simulink model "gm_lookupTable"  (R2019b)
settings: Solver=FixedStepAuto  StartTime=0.0  StopTime=0.01  RelTol=1e-3
libraries: hdlsllib x1
settings Model: Creator=bwieczorek  LastModifiedBy=bwieczorek
settings OptimizationCC: BlockReduction=off  ConditionallyExecuteInputs=off
settings DebuggingCC: SignalRangeChecking=warning  InheritedTsInSrcMsg=none

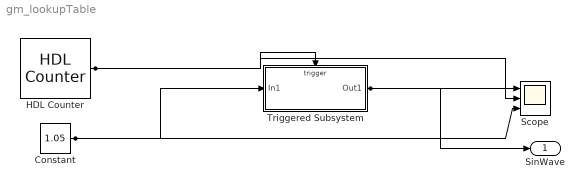
== system gm_lookupTable ==
  Constant : Constant  Value=1.05  OutDataTypeStr=fixdt(1,18,8)  SampleTime=1e-6
  HDL Counter : hdlsllib/Sources/HDL Counter  CountType=Count limited  CountInit=0  CountStep=1  CountMax=1  CountFromType=Initial value  CountFrom=0  CountResetPort=off  CountLoadPort=off  CountEnbPort=off  CountDirPort=off  CountDataType=Unsigned  CountWordLen=1  CountFracLen=0  CountSampTime=1e-6
      settings: SourceProductName=Simulink
  Scope : Scope  NumInputPorts=3
  Triggered Subsystem : Subsystem
  SinWave : Outport  VectorParamsAs1DForOutWhenUnconnected=off
  wires:
  Constant/1 -> Scope/3, Triggered Subsystem/1(In1)
  HDL Counter/1 -> Scope/2, Triggered Subsystem/Trigger
  Triggered Subsystem/1(Out1) -> Scope/1, SinWave/1

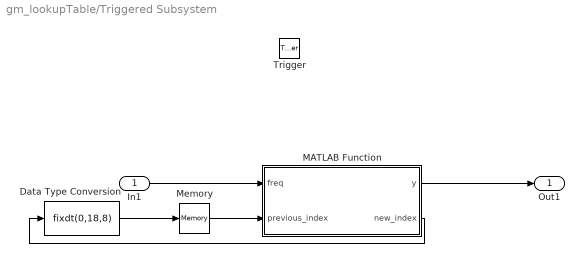
== system gm_lookupTable/Triggered Subsystem ==
  In1 : Inport  OutDataTypeStr=fixdt(1, 18, 8)  PortDimensions=1
  Trigger : TriggerPort  VariantControl=(inherit)  InitialTriggerSignalState=zero  PortDimensions=1  OutDataTypeStr=fixdt(0, 1, 0)
  Data Type Conversion : DataTypeConversion  OutDataTypeStr=fixdt(0,18,8)
  MATLAB Function : Subsystem
  Memory : Memory  InheritSampleTime=on
  Out1 : Outport  InitialOutput=0
  wires:
  In1/1 -> MATLAB Function/1(freq)
  Data Type Conversion/1 -> Memory/1
  MATLAB Function/1(y) -> Out1/1
  MATLAB Function/2(new_index) -> Data Type Conversion/1
  Memory/1 -> MATLAB Function/2(previous_index)

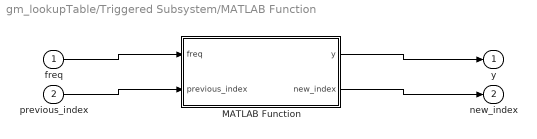
== system gm_lookupTable/Triggered Subsystem/MATLAB Function ==
  freq : Inport  OutDataTypeStr=fixdt(1, 18, 8)  PortDimensions=1
  previous_index : Inport  Port=2  OutDataTypeStr=fixdt(0, 18, 8)  PortDimensions=1
  MATLAB Function : MATLAB Function  TreatAsAtomicUnit=on
  y : Outport  InitialOutput=0  VectorParamsAs1DForOutWhenUnconnected=off
  new_index : Outport  Port=2  InitialOutput=0
  wires:
  freq/1 -> MATLAB Function/1(freq)
  previous_index/1 -> MATLAB Function/2(previous_index)
  MATLAB Function/1(y) -> y/1
  MATLAB Function/2(new_index) -> new_index/1

== matlab function gm_lookupTable/Triggered Subsystem/MATLAB Function/MATLAB Function ==
  data: freq input; y output; previous_index input fixdt(0,18,8); new_index output fixdt(0,19,8)
function [y, new_index]= fcn(freq, previous_index)
%#codegen
loader = coder.load('tableSin.mat');
table = loader.tableSin;
new_index = fi(previous_index + freq, 0, 19, 8);
if(new_index >= 256)
new_index = fi(new_index - fi(256,0,9,0),0,19,8);    
end
if(mod(new_index, fi(1,0,1,0)) == 0 )
y = fi(table((mod(new_index,fi(256,0,9,0)))+1),1,18,17);
else
index_floor = floor(new_index);
if(index_floor == 255)
index_ceil = fi(0,0,12,0); 
else
index_ceil = ceil(new_index);    
end
sin_floor = table(index_floor+1);
sin_ceil = table(index_ceil+1);
a = sin_ceil - sin_floor;
y = fi(a*mod(new_index,fi(1,0,1,0)) + sin_floor, 1, 18, 17);
end
